simulink model "MMC_avg_v3"  (R2022b)
settings: Solver=VariableStepAuto  StartTime=0.0  StopTime=0.6  RelTol=1e-3
undefined symbols (not defined in the file or in its folder): DiscIntNeverNeededParam, plecs, Ts
libraries: simulink x4
settings Model: Creator=Asus  LastModifiedBy=ben19
settings DebuggingCC: UnconnectedInputMsg=warning  UnconnectedOutputMsg=warning  UnconnectedLineMsg=warning
settings ModelReferenceCC: EnableRefExpFcnMdlSchedulingChecks=on
settings RTWCC: DLArmComputeVersion=19.05

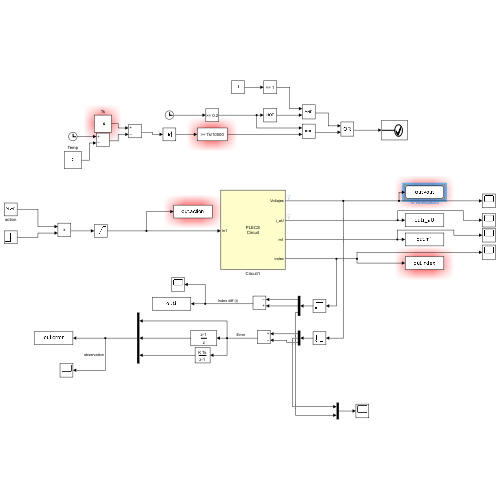
[thumbnail: Simulink's stored preview of the top-level diagram]
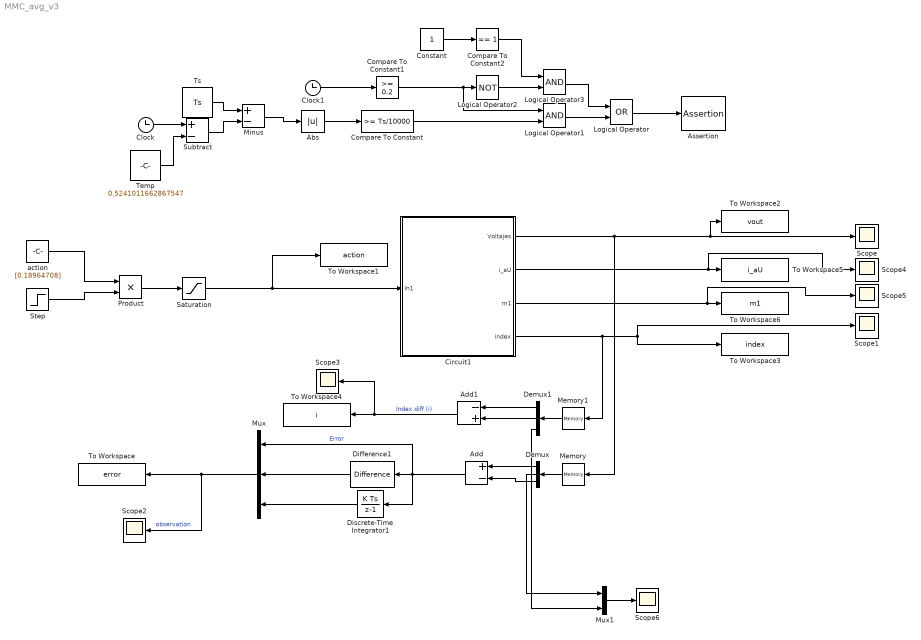
== system MMC_avg_v3 ==
  Abs : Abs  SaturateOnIntegerOverflow=off
  Add : Sum  Inputs=+-
  Add1 : Sum  Inputs=-+
  Assertion : Assertion  AssertionFailFcn=set_param(bdroot,'SimulationCommand','pause')  StopWhenAssertionFail=off
  Circuit1 : Subsystem  LoadFcn=plecs('sl', 200);  InitFcn=plecs('sl', 214);  StartFcn=plecs('sl', 208);  StopFcn=plecs('sl', 209);  mask(PlecsCircuit){PLECSData=<binary blob, 67180 chars, not shown>}
      mask prompts: PLECSData "PLECS Data (Do not delete or modify!)"
      mask init:
      | % PLACE CUSTOM INITIALIZATIONS ABOVE
      | % DO NOT REMOVE
      | plecs('sl', 215);
      | % DO NOT REMOVE
      settings: CopyFcn=plecs('sl', 203);  DeleteFcn=plecs('sl', 205);  UndoDeleteFcn=plecs('sl', 206);  PreSaveFcn=plecs('sl', 211);  PostSaveFcn=plecs('sl', 201);  NameChangeFcn=plecs('sl', 210);  DestroyFcn=plecs('sl', 207);  PreCopyFcn=plecs('sl', 216);  OpenFcn=plecs('sl', 202);  ErrorFcn=plerrorfcn
      mask Help: web(['file:///' fullfile(plecsdoc, 'creatingacircuit.html')])
      mask Display: disp('PLECS\nCircuit')
  Clock : Clock
  Clock1 : Clock
  Compare To Constant : simulink/Logic and Bit Operations/Compare To Constant  relop=>=  const=Ts/10000  OutDataTypeStr=boolean
  Compare To Constant1 : simulink/Logic and Bit Operations/Compare To Constant  relop=>=  const=0.2  OutDataTypeStr=boolean
  Compare To Constant2 : simulink/Logic and Bit Operations/Compare To Constant  relop===  const=1  OutDataTypeStr=boolean
  Constant : Constant
  Demux : Demux  Outputs=3
  Demux1 : Demux  Outputs=3
  Difference1 : simulink/Discrete/Difference  ICPrevInput=0.0  OutMin=[]  OutMax=[]  OutDataType=fixdt(1, 16)  OutScaling=2^-10  DoSatur=off
  Discrete-Time Integrator1 : DiscreteIntegrator  SampleTime=-1  ICPrevOutput=DiscIntNeverNeededParam  ICPrevScaledInput=DiscIntNeverNeededParam
  Logical Operator : Logic  Operator=OR  AllPortsSameDT=off  OutDataTypeStr=boolean
  Logical Operator1 : Logic  AllPortsSameDT=off  OutDataTypeStr=boolean
  Logical Operator2 : Logic  Operator=NOT  AllPortsSameDT=off  OutDataTypeStr=boolean
  Logical Operator3 : Logic  AllPortsSameDT=off  OutDataTypeStr=boolean
  Memory : Memory
  Memory1 : Memory
  Minus : Sum  Inputs=+-
  Mux : Mux  Inputs=3
  Mux1 : Mux  Inputs=2
  Product : Product
  Saturation : Saturate  UpperLimit=50  LowerLimit=-50
  Scope{,1..6} (7 alike) : Scope
  Step : Step  Time=0.2  SampleTime=0
  Subtract : Sum  Inputs=+-
  Temp : Constant  Value=0.5241011662867547
  To Workspace : ToWorkspace  VariableName=error  SampleTime=-1
      settings: Save2DSignal=2-D array (concatenate along first dimension)
  To Workspace1 : ToWorkspace  VariableName=action  SampleTime=Ts
      settings: Save2DSignal=2-D array (concatenate along first dimension)
  To Workspace2 : ToWorkspace  VariableName=vout  SaveFormat=Timeseries  SampleTime=Ts
      settings: Save2DSignal=2-D array (concatenate along first dimension)
  To Workspace3 : ToWorkspace  VariableName=index  SampleTime=Ts
      settings: Save2DSignal=2-D array (concatenate along first dimension)
  To Workspace4 : ToWorkspace  VariableName=i  SampleTime=-1
      settings: Save2DSignal=2-D array (concatenate along first dimension)
  To Workspace5 : ToWorkspace  VariableName=i_aU  SampleTime=-1
      settings: Save2DSignal=2-D array (concatenate along first dimension)
  To Workspace6 : ToWorkspace  VariableName=m1  SampleTime=-1
      settings: Save2DSignal=2-D array (concatenate along first dimension)
  Ts : Constant  Value=Ts
  action : Constant  Value=[0.18964708]
  wires:
  Circuit1/1(Voltajes) -> Scope/1, To Workspace2/1, Memory/1
  Circuit1/4(index) -> Memory1/1, To Workspace3/1, Scope1/1
  Memory/1 -> Demux/1
  Demux/1 -> Add/1
  Add/1 -> Discrete-Time Integrator1/1, Difference1/1, Mux/1  "Error"
  Discrete-Time Integrator1/1 -> Mux/3
  Demux/3 -> Add/2
  Mux/1 -> To Workspace/1, Scope2/1  "observation"
  Memory1/1 -> Demux1/1
  Demux1/2 -> Add1/2
  Demux1/1 -> Add1/1
  Add1/1 -> To Workspace4/1, Scope3/1  "Index diff (i)"
  action/1 -> Product/1
  Step/1 -> Product/2
  Saturation/1 -> Circuit1/1(In1), To Workspace1/1
  Product/1 -> Saturation/1
  Clock/1 -> Subtract/1
  Temp/1 -> Subtract/2
  Ts/1 -> Minus/1
  Subtract/1 -> Minus/2
  Circuit1/2(i_aU) -> Scope4/1, To Workspace5/1
  Circuit1/3(m1) -> Scope5/1, To Workspace6/1
  Minus/1 -> Abs/1
  Abs/1 -> Compare To Constant/1
  Logical Operator/1 -> Assertion/1
  Clock1/1 -> Compare To Constant1/1
  Compare To Constant/1 -> Logical Operator1/2
  Compare To Constant1/1 -> Logical Operator2/1, Logical Operator1/1
  Logical Operator1/1 -> Logical Operator/2
  Constant/1 -> Compare To Constant2/1
  Logical Operator2/1 -> Logical Operator3/2
  Compare To Constant2/1 -> Logical Operator3/1
  Logical Operator3/1 -> Logical Operator/1
  Difference1/1 -> Mux/2
  Demux1/3 -> Mux1/2
  Demux/2 -> Mux1/1
  Mux1/1 -> Scope6/1

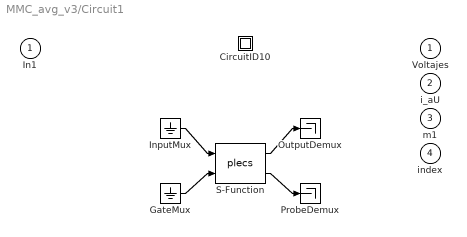
== system MMC_avg_v3/Circuit1 ==
  In1 : Inport  PortDimensions=1
  " CircuitID10 " : Subsystem
  " GateMux " : Ground
  " InputMux " : Ground
  " OutputDemux " : Terminator
  " ProbeDemux " : Terminator
  " S-Function " : S-Function  FunctionName=plecs  SFunctionDeploymentMode=off  EnableBusSupport=off
  Voltajes : Outport  PortDimensions=3
  i_aU : Outport  Port=2  PortDimensions=1
  m1 : Outport  Port=3  PortDimensions=1
  index : Outport  Port=4  PortDimensions=3
  wires:
  " InputMux "/1 -> " S-Function "/1
  " GateMux "/1 -> " S-Function "/2
  " S-Function "/1 -> " OutputDemux "/1
  " S-Function "/2 -> " ProbeDemux "/1

== system MMC_avg_v3/Circuit1/ CircuitID10  ==
